simulink model "ev"  (R2021a)
settings: Solver=ode4  StartTime=0  StopTime=1082  FixedStep=sim_dt  RelTol=1e-3
model workspace (MAT data in the model file):
  T_eff_bp = [-270; -210; -150; -90; -30; 30; 90; 150; 210; 270]
  T_eff_bp_2 = [-270; -210; -150; -90; -30; 30; 90; 150; 210; 270]
  losses_table = [108927.107777 7820.2782368 7820.17609997 7820.2782368 7820.2782368 7820.2782368 7820.2782368 7820.26172359 7820.2782368 9345.38006027 108927.107777 7820.2782368 ... (100 elements, 10x10)]
  losses_table_2 = [108927.107777 7820.2782368 7820.17609997 7820.2782368 7820.2782368 7820.2782368 7820.2782368 7820.26172359 7820.2782368 9345.38006027 108927.107777 7820.2782368 ... (100 elements, 10x10)]
  w_eff_bp = [0; 888.888888889; 1777.77777778; 2666.66666667; 3555.55555556; 4444.44444444; 5333.33333333; 6222.22222222; 7111.11111111; 8000]
  w_eff_bp_2 = [0; 888.888888889; 1777.77777778; 2666.66666667; 3555.55555556; 4444.44444444; 5333.33333333; 6222.22222222; 7111.11111111; 8000]
undefined symbols (not defined in the file): Af, alpha, Bt, C, C_fa, C_free, C_sa_bat, C_sa_uc, Cd, Cmax, Continuous, Crr, DoD, effi, etaFD, etaG, FD, G, gear, Iucmax, m, M1m, M2m, Max, npar, npar_free, npara, nparf, nparfa, nparsa_bat, nparsa_UC, nser, nser_free, nserfa, nsersa_bat, nsersa_UC, Qbat, regenmax, Ri_BP, RL, ro, Rsc, Rsc_A, Rsc_F, Rsc_sa_bat, Rsc_sa_uc, rw, sim_dt, SOC_BP, SoCbatmax, SoCbatmin, SoCucmax, SoCucmin, speed, torque, VinBat, Voc_BP, Vuc, Vuc_fa, Vuc_free ... (+2)
libraries: autolibshared x41, simulink x26, autolibdcdc x13, autolibdatasheetbattery x7, autolibmappedmotor x6, fl_lib x3, nesl_utility x3, spsSupercapacitorLib x3, pid_lib x1
(part 11 of 18)

== system ev/Tesis/HESS/Full_active/Subsystem ==
  power : Inport
  motor_pwr_contr : Inport  Port=2
  1-D Lookup Table : Lookup_n-D  NumberOfTableDimensions=1  BreakpointsForDimension1=Continuous(:,1)  Table=Continuous(:,2)  InternalRulePriority=Speed  RndMeth=Simplest  InputSameDT=on
  1-D Lookup Table2 : Lookup_n-D  NumberOfTableDimensions=1  BreakpointsForDimension1=Continuous(:,1)  Table=-Continuous(:,2)  InternalRulePriority=Speed  RndMeth=Simplest  InputSameDT=on
  Constant : Constant  Value=0
  Constant1 : Constant
  Divide1 : Product  Inputs=**
  Divide2 : Product  Inputs=**
  Divide3 : Product  Inputs=*/
  Gain2 : Gain  Gain=30/pi
  Gain4 : Gain  Gain=0.95
  Gain5 : Gain  Gain=1/rw
  Gain6 : Gain  Gain=1/0.95
  Manual Switch : ManualSwitch  CurrentSetting=0
  Saturation Dynamic : simulink/Discontinuities/Saturation Dynamic  OutMin=[]  OutMax=[]  OutDataTypeStr=Inherit: Same as second input  OutDataType=fixdt(1, 16)  OutScaling=2^-10  DoSatur=off
  Scope : Scope
  Scope1 : Scope
  Switch : Switch  Criteria=u2 ~= 0
  Switch1 : Switch
  Switch2 : Switch  Criteria=u2 ~= 0
  motor speed estimation : Subsystem
  Out1 : Outport
  tag scope: spd_real=global, trq_real=global
  wires:
  motor_pwr_contr/1 -> Switch1/2
  Gain4/1 -> Divide1/1  "breaking torque"
  [gear_ratio] -> Divide1/2
  Divide1/1 -> Switch1/1
  Switch1/1 -> [trq_real], Gain5/1  "motor torque"
  Gain5/1 -> Out1/1  "FORCE"
  [gear_ratio] -> Divide2/2
  Gain6/1 -> Divide2/1  "motor_torque"
  Divide2/1 -> Switch1/3
  Divide3/1 -> Switch/1, Scope/1  "torque"
  power/1 -> Divide3/1  "power"
  Gain2/1 -> 1-D Lookup Table2/1, 1-D Lookup Table/1
  1-D Lookup Table/1 -> Saturation Dynamic/1
  1-D Lookup Table2/1 -> Saturation Dynamic/3
  Saturation Dynamic/1 -> Gain4/1, Gain6/1
  Switch/1 -> Saturation Dynamic/2
  Constant/1 -> Switch/3
  motor speed estimation/1(motor angular speed) -> Manual Switch/2  "motor angular speed required"
  Manual Switch/1 -> [spd_real], Scope1/1, Gain2/1, Switch2/1, Switch2/2, Switch/2
  [mtr_speed] -> Manual Switch/1
  [Veh_real_FA] -> motor speed estimation/1(vel_m/s)
  Switch2/1 -> Divide3/2
  Constant1/1 -> Switch2/3
